simulink model "Inbuild_PID_final"  (R2021a)
settings: Solver=FixedStepAuto  StartTime=0.0  StopTime=inf  RelTol=1e-3
model workspace (MAT data in the model file):
  SL_ROS_VariableLengthArrays_MaxSizes.CommonInfo.ArrayTruncateAction = 'EmitWarning'
  SL_ROS_VariableLengthArrays_MaxSizes.MsgTypeMap = containers.Map
  SL_ROS_VariableLengthArrays_MaxSizes.MsgTypeMap.serialization.keys = {'sensor_msgs/JointState'}
  SL_ROS_VariableLengthArrays_MaxSizes.MsgTypeMap.serialization.values{1}(1).PropertyName = 'Effort'
  SL_ROS_VariableLengthArrays_MaxSizes.MsgTypeMap.serialization.values{1}(1).DataType = 'double'
  SL_ROS_VariableLengthArrays_MaxSizes.MsgTypeMap.serialization.values{1}(1).MaxLength = 128
  SL_ROS_VariableLengthArrays_MaxSizes.MsgTypeMap.serialization.values{1}(2).PropertyName = 'Name'
  SL_ROS_VariableLengthArrays_MaxSizes.MsgTypeMap.serialization.values{1}(2).DataType = 'std_msgs/String'
  SL_ROS_VariableLengthArrays_MaxSizes.MsgTypeMap.serialization.values{1}(2).MaxLength = 16
  SL_ROS_VariableLengthArrays_MaxSizes.MsgTypeMap.serialization.values{1}(3).PropertyName = 'Position'
  SL_ROS_VariableLengthArrays_MaxSizes.MsgTypeMap.serialization.values{1}(3).DataType = 'double'
  SL_ROS_VariableLengthArrays_MaxSizes.MsgTypeMap.serialization.values{1}(3).MaxLength = 3
  SL_ROS_VariableLengthArrays_MaxSizes.MsgTypeMap.serialization.values{1}(4).PropertyName = 'Velocity'
  SL_ROS_VariableLengthArrays_MaxSizes.MsgTypeMap.serialization.values{1}(4).DataType = 'double'
  SL_ROS_VariableLengthArrays_MaxSizes.MsgTypeMap.serialization.values{1}(4).MaxLength = 128
  SL_ROS_VariableLengthArrays_MaxSizes.MsgTypeMap.serialization.uniformity = 0
  SL_ROS_VariableLengthArrays_MaxSizes.MsgTypeMap.serialization.keyType = 'char'
  SL_ROS_VariableLengthArrays_MaxSizes.MsgTypeMap.serialization.valueType = 'any'
libraries: robotlib x6
settings Model: Creator=Dr.Saraf  LastModifiedBy=reaperj
settings SolverCC: AlgebraicLoopSolver=TrustRegion
settings OptimizationCC: EnhancedBackFolding=on  PassReuseOutputArgsAs=Individual arguments  ZeroExternalMemoryAtStartup=off  ZeroInternalMemoryAtStartup=off  MaxStackSize=64  OptimizeBlockOrder=speed  DifferentSizesBufferReuse=on  OptimizationCustomize=off  EfficientTunableParamExpr=on
settings DebuggingCC: ParameterTunabilityLossMsg=error  SFMachineParentedDataDiag=warning
settings HardwareCC: ProdBitPerPointer=32  ProdBitPerSizeT=32  ProdBitPerPtrDiffT=32  ProdLargestAtomicFloat=None  ProdIntDivRoundTo=Undefined  ProdEndianess=Unspecified  ProdWordSize=32  ProdHWDeviceType=Generic->Unspecified (assume 32-bit Generic)  UseEmbeddedCoderFeatures=off  UseSimulinkCoderFeatures=off
settings SFSimCC: MATLABDynamicMemAlloc=off
settings RTWCC: SystemTargetFile=ert.tlc  HardwareBoard=Robot Operating System (ROS)  TLCOptions="-aInlineSetEventsForThisBaseRateFcn=TLC_FALSE -aSuppressMultiTaskScheduler=TLC_FALSE  -aRateBasedStepFcn=0"  TemplateMakefile=ert_default_tmf  Toolchain=Catkin  TargetLang=C++
settings CodeAppCC: ForceParamTrailComments=on  IgnoreCustomStorageClasses=off  OperatorAnnotations=on  SimulinkDataObjDesc=on  SFDataObjDesc=on  InsertBlockDesc=on
settings ERTTargetCC: SupportNonInlinedSFcns=on

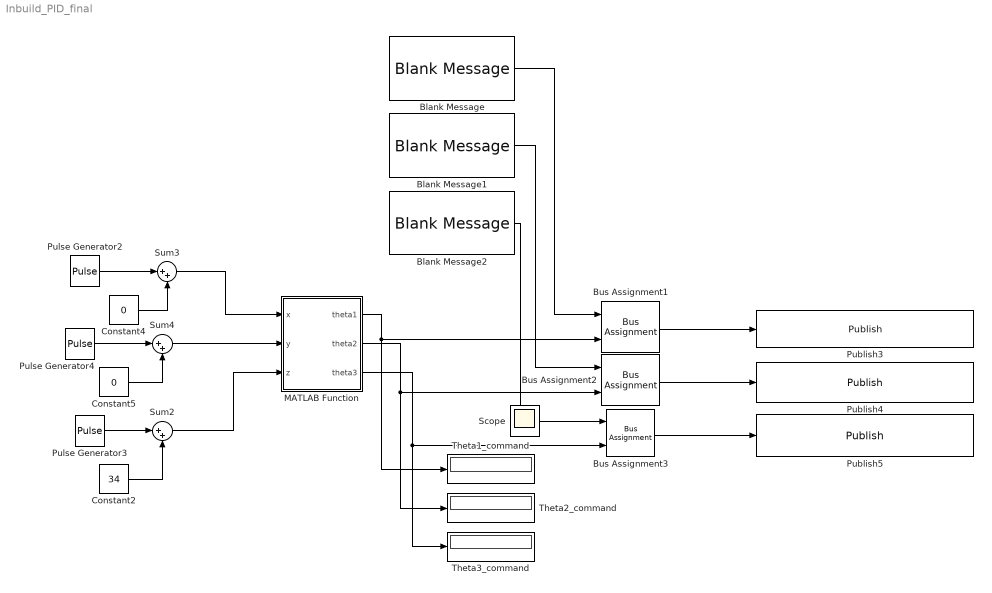
== system Inbuild_PID_final ==
  Blank Message : robotlib/Blank Message  messageClass=Message  entityType=std_msgs/Float64  messageType=std_msgs/Float64  SampleTime=.1  legacyBusStruct=off
  Blank Message1 : robotlib/Blank Message  messageClass=Message  entityType=std_msgs/Float64  messageType=std_msgs/Float64  SampleTime=.1  legacyBusStruct=off
  Blank Message2 : robotlib/Blank Message  messageClass=Message  entityType=std_msgs/Float64  messageType=std_msgs/Float64  SampleTime=.1  legacyBusStruct=off
  Bus Assignment1 : BusAssignment  AssignedSignals=Data
  Bus Assignment2 : BusAssignment  AssignedSignals=Data
  Bus Assignment3 : BusAssignment  AssignedSignals=Data
  Constant2 : Constant  Value=34  SampleTime=.1
  Constant4 : Constant  Value=0  SampleTime=.1
  Constant5 : Constant  Value=0  SampleTime=.1
  MATLAB Function : MATLAB Function  TreatAsAtomicUnit=on
  Publish3 : robotlib/Publish  topicSource=Select from ROS network  topic=/iiwa/joint1_position_controller/command  messageType=std_msgs/Float64  legacyBusStruct=off  messageQueueLength=1
  Publish4 : robotlib/Publish  topicSource=Select from ROS network  topic=/iiwa/joint2_position_controller/command  messageType=std_msgs/Float64  legacyBusStruct=off  messageQueueLength=1
  Publish5 : robotlib/Publish  topicSource=Select from ROS network  topic=/iiwa/joint4_position_controller/command  messageType=std_msgs/Float64  legacyBusStruct=off  messageQueueLength=1
  Pulse Generator2 : DiscretePulseGenerator  PulseType=Time based  Amplitude=50  Period=300  PulseWidth=50
  Pulse Generator3 : DiscretePulseGenerator  PulseType=Time based  Amplitude=40  Period=300  PulseWidth=50  PhaseDelay=150
  Pulse Generator4 : DiscretePulseGenerator  PulseType=Time based  Amplitude=-50  Period=300  PulseWidth=50  PhaseDelay=150
  Sum2 : Sum  Inputs=|++
  Sum3 : Sum  Inputs=|++
  Sum4 : Sum  Inputs=|++
  Theta1_command : Display
  Theta2_command : Display
  Theta3_command : Display
  Scope : Scope
  wires:
  Bus Assignment1/1 -> Publish3/1
  Blank Message/1 -> Bus Assignment1/1
  Blank Message1/1 -> Bus Assignment2/1
  Bus Assignment2/1 -> Publish4/1
  Blank Message2/1 -> Bus Assignment3/1
  Bus Assignment3/1 -> Publish5/1
  MATLAB Function/1(theta1) -> Bus Assignment1/2, Theta1_command/1
  MATLAB Function/2(theta2) -> Theta2_command/1, Bus Assignment2/2
  MATLAB Function/3(theta3) -> Theta3_command/1, Bus Assignment3/2
  Sum4/1 -> MATLAB Function/2(y)
  Constant2/1 -> Sum2/2
  Sum2/1 -> MATLAB Function/3(z)
  Constant5/1 -> Sum4/2
  Pulse Generator4/1 -> Sum4/1
  Sum3/1 -> MATLAB Function/1(x)
  Pulse Generator3/1 -> Sum2/1
  Constant4/1 -> Sum3/2
  Pulse Generator2/1 -> Sum3/1

== matlab function Inbuild_PID_final/MATLAB Function ==
  data: x input; theta1 output; y input; z input; theta2 output; theta3 output
%% Inverse Kinematics
function [theta1, theta2, theta3] = invk(x,y,z)

a1 = 34; a2 = 40; a3 = 52.6;

r1 = sqrt(x^2 + y^2);
r2 = a1 - z;
if(r1== 0 && r2>=0)
    phi2 = pi/2;
elseif(r1== 0 && r2<0)
    phi2 = -pi/2;
else
    phi2 = atan(r2/r1);
end

r3 = sqrt(r1^2 + r2^2);
if(r3== 0)
    phi1 = 0;
else
    phi1 = acos((a3^2 - a2^2 - r3^2)/(-2*a2*r3));
end

phi3 = acos((r3^2 - a2^2 - a3^2)/(-2*a2*a3));

if(y == 0)
    theta1 = 0 ;
else
    theta1 = atan(y/x);
end

theta2 = phi2 - phi1 ;
theta3 = - pi + phi3;

theta1 = theta1 + (pi/2) ;
theta2 = theta2 + (pi/2);


end
